simulink model "BME331Lab3SimModel"  (R2022b)
settings: Solver=VariableStepAuto  StartTime=0.0  StopTime=10.0  RelTol=1e-3
undefined symbols (not defined in the file or in its folder): g, h, l, m
settings Model: Creator=ihass  LastModifiedBy=ihass

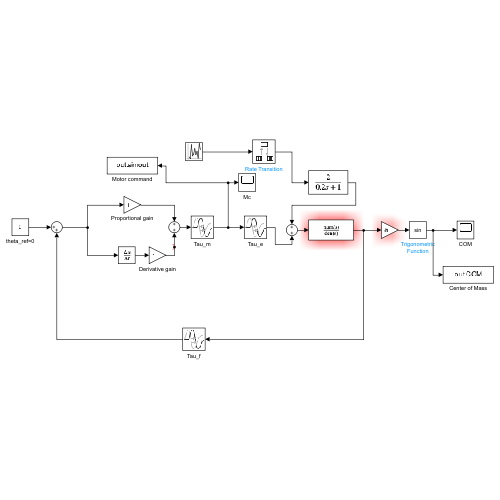
[thumbnail: Simulink's stored preview of the top-level diagram]
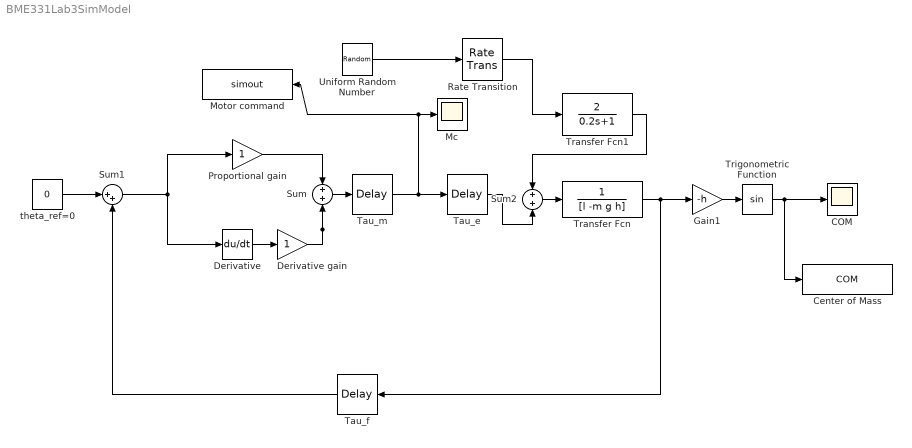
== system BME331Lab3SimModel ==
  COM : Scope
  Center of Mass : ToWorkspace  VariableName=COM  SaveFormat=Timeseries  SampleTime=-1
  Derivative : Derivative
  Derivative gain : Gain
  Gain1 : Gain  Gain=-h
  Mc : Scope
  Motor command : ToWorkspace  VariableName=simout  SaveFormat=Timeseries  SampleTime=-1
  Proportional gain : Gain
  Rate Transition : RateTransition
  Sum : Sum  Inputs=+|+
  Sum1 : Sum  Inputs=|++
  Sum2 : Sum  Inputs=+|+
  Tau_e : TransportDelay  DelayTime=0.01
  Tau_f : TransportDelay  DelayTime=0.04
  Tau_m : TransportDelay
  Transfer Fcn : TransferFcn  Denominator=[l -m g h]
  Transfer Fcn1 : TransferFcn  Numerator=[2]  Denominator=[0.2 1]
  Trigonometric Function : Trigonometry
  Uniform Random Number : UniformRandomNumber  SampleTime=0.1
  theta_ref=0 : Constant  Value=0
  wires:
  Derivative gain/1 -> Sum/2
  Proportional gain/1 -> Sum/1
  Derivative/1 -> Derivative gain/1
  Tau_f/1 -> Sum1/2
  Transfer Fcn/1 -> Tau_f/1, Gain1/1
  Gain1/1 -> Trigonometric Function/1
  Trigonometric Function/1 -> Center of Mass/1, COM/1
  Sum/1 -> Tau_m/1
  Sum1/1 -> Proportional gain/1, Derivative/1
  theta_ref=0/1 -> Sum1/1
  Tau_m/1 -> Motor command/1, Mc/1, Tau_e/1
  Uniform Random Number/1 -> Rate Transition/1
  Rate Transition/1 -> Transfer Fcn1/1
  Tau_e/1 -> Sum2/2
  Transfer Fcn1/1 -> Sum2/1
  Sum2/1 -> Transfer Fcn/1
